simulink model "laba_2"  (R2020b)
settings: Solver=VariableStepAuto  StartTime=0.0  StopTime=15  RelTol=1e-3
settings Model: Creator=vak90  LastModifiedBy=Mi-Mi-Mishka
settings DebuggingCC: ArithmeticOperatorsInVariantConditions=warning
settings SFSimCC: CustomCodeUndefinedFunction=UseInterfaceOnly

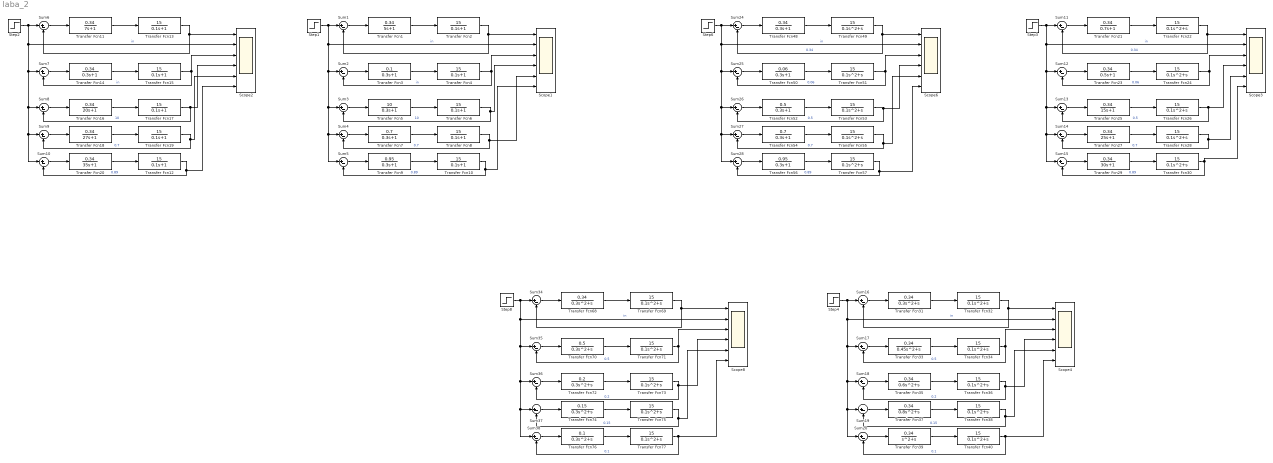
== system laba_2 ==
  Scope{1..4,6,8} (6 alike) : Scope  NumInputPorts=6
  Step{1..4,6,8} (6 alike) : Step  Time=0.1  SampleTime=0
  Sum{1..20,24..28,34..38} (30 alike) : Sum  Inputs=|+-
  Transfer Fcn1 : TransferFcn  Numerator=[0.34]  Denominator=[5 1]
  Transfer Fcn{2,4,6,8,10,12..13,15,17,19} (10 alike) : TransferFcn  Numerator=[15]  Denominator=[0.1 1 ]
  Transfer Fcn11 : TransferFcn  Numerator=[0.34]  Denominator=[7 1]
  Transfer Fcn14 : TransferFcn  Numerator=[0.34]  Denominator=[0.3 1]
  Transfer Fcn16 : TransferFcn  Numerator=[0.34]  Denominator=[20 1]
  Transfer Fcn18 : TransferFcn  Numerator=[0.34]  Denominator=[27 1]
  Transfer Fcn20 : TransferFcn  Numerator=[0.34]  Denominator=[35 1]
  Transfer Fcn21 : TransferFcn  Numerator=[0.34]  Denominator=[0.7 1]
  Transfer Fcn{22,24,26,28,30,32,34,36,38,40,49,51,53,55,57,69,71,73,75,77} (20 alike) : TransferFcn  Numerator=[15]  Denominator=[0.1 1 0]
  Transfer Fcn23 : TransferFcn  Numerator=[0.34]  Denominator=[0.5 1]
  Transfer Fcn25 : TransferFcn  Numerator=[0.34]  Denominator=[15 1]
  Transfer Fcn27 : TransferFcn  Numerator=[0.34]  Denominator=[25 1]
  Transfer Fcn29 : TransferFcn  Numerator=[0.34]  Denominator=[30 1]
  Transfer Fcn3 : TransferFcn  Numerator=[0.1]  Denominator=[0.3 1]
  Transfer Fcn31 : TransferFcn  Numerator=[0.34]  Denominator=[0.3 1 0]
  Transfer Fcn33 : TransferFcn  Numerator=[0.34]  Denominator=[0.45 1 0]
  Transfer Fcn35 : TransferFcn  Numerator=[0.34]  Denominator=[0.6 1 0]
  Transfer Fcn37 : TransferFcn  Numerator=[0.34]  Denominator=[0.8 1 0]
  Transfer Fcn39 : TransferFcn  Numerator=[0.34]  Denominator=[1 1 0]
  Transfer Fcn48 : TransferFcn  Numerator=[0.34]  Denominator=[0.3 1]
  Transfer Fcn5 : TransferFcn  Numerator=[10]  Denominator=[0.3 1]
  Transfer Fcn50 : TransferFcn  Numerator=[0.06]  Denominator=[0.3 1]
  Transfer Fcn52 : TransferFcn  Numerator=[0.5]  Denominator=[0.3 1]
  Transfer Fcn54 : TransferFcn  Numerator=[0.7]  Denominator=[0.3 1]
  Transfer Fcn56 : TransferFcn  Numerator=[0.95]  Denominator=[0.3 1]
  Transfer Fcn68 : TransferFcn  Numerator=[0.34]  Denominator=[0.3 1 0]
  Transfer Fcn7 : TransferFcn  Numerator=[0.7]  Denominator=[0.3 1]
  Transfer Fcn70 : TransferFcn  Numerator=[0.5]  Denominator=[0.3 1 0]
  Transfer Fcn72 : TransferFcn  Numerator=[0.2]  Denominator=[0.3 1 0]
  Transfer Fcn74 : TransferFcn  Numerator=[0.15]  Denominator=[0.3 1 0]
  Transfer Fcn76 : TransferFcn  Numerator=[0.1]  Denominator=[0.3 1 0]
  Transfer Fcn9 : TransferFcn  Numerator=[0.95]  Denominator=[0.3 1]
  wires:
  Step6/1 -> Sum28/1, Sum27/1, Sum26/1, Sum25/1, Scope6/2, Sum24/1  "in"
  Sum24/1 -> Transfer Fcn48/1
  Transfer Fcn48/1 -> Transfer Fcn49/1
  Transfer Fcn49/1 -> Sum24/2, Scope6/1  "0.34"
  Sum25/1 -> Transfer Fcn50/1
  Transfer Fcn50/1 -> Transfer Fcn51/1
  Sum26/1 -> Transfer Fcn52/1
  Transfer Fcn52/1 -> Transfer Fcn53/1
  Sum27/1 -> Transfer Fcn54/1
  Transfer Fcn54/1 -> Transfer Fcn55/1
  Sum28/1 -> Transfer Fcn56/1
  Transfer Fcn56/1 -> Transfer Fcn57/1
  Transfer Fcn51/1 -> Sum25/2, Scope6/3  "0.06"
  Transfer Fcn53/1 -> Scope6/4, Sum26/2  "0.5"
  Transfer Fcn55/1 -> Scope6/5, Sum27/2  "0.7"
  Transfer Fcn57/1 -> Scope6/6, Sum28/2  "0.89"
  Transfer Fcn68/1 -> Transfer Fcn69/1
  Transfer Fcn69/1 -> Sum34/2, Scope8/1
  Sum34/1 -> Transfer Fcn68/1
  Transfer Fcn73/1 -> Scope8/4, Sum36/2  "0.2"
  Step8/1 -> Sum38/1, Sum37/1, Sum36/1, Sum35/1, Scope8/2, Sum34/1  "in"
  Transfer Fcn71/1 -> Sum35/2, Scope8/3  "0.5"
  Transfer Fcn77/1 -> Scope8/6, Sum38/2  "0.1"
  Transfer Fcn75/1 -> Scope8/5, Sum37/2  "0.15"
  Sum35/1 -> Transfer Fcn70/1
  Transfer Fcn70/1 -> Transfer Fcn71/1
  Sum36/1 -> Transfer Fcn72/1
  Transfer Fcn72/1 -> Transfer Fcn73/1
  Sum37/1 -> Transfer Fcn74/1
  Transfer Fcn74/1 -> Transfer Fcn75/1
  Sum38/1 -> Transfer Fcn76/1
  Transfer Fcn76/1 -> Transfer Fcn77/1
  Sum4/1 -> Transfer Fcn7/1
  Transfer Fcn1/1 -> Transfer Fcn2/1
  Transfer Fcn3/1 -> Transfer Fcn4/1
  Transfer Fcn10/1 -> Scope1/6, Sum5/2  "0.89"
  Transfer Fcn2/1 -> Sum1/2, Scope1/1
  Transfer Fcn7/1 -> Transfer Fcn8/1
  Step1/1 -> Sum5/1, Sum4/1, Sum3/1, Sum2/1, Scope1/2, Sum1/1  "in"
  Transfer Fcn6/1 -> Scope1/4, Sum3/2  "10"
  Sum2/1 -> Transfer Fcn3/1
  Sum5/1 -> Transfer Fcn9/1
  Transfer Fcn8/1 -> Scope1/5, Sum4/2  "0.7"
  Sum3/1 -> Transfer Fcn5/1
  Sum1/1 -> Transfer Fcn1/1
  Transfer Fcn5/1 -> Transfer Fcn6/1
  Transfer Fcn9/1 -> Transfer Fcn10/1
  Transfer Fcn4/1 -> Sum2/2, Scope1/3  "in"
  Transfer Fcn20/1 -> Transfer Fcn12/1
  Transfer Fcn13/1 -> Sum6/2, Scope2/1
  Sum8/1 -> Transfer Fcn16/1
  Sum9/1 -> Transfer Fcn18/1
  Sum6/1 -> Transfer Fcn11/1
  Transfer Fcn16/1 -> Transfer Fcn17/1
  Sum7/1 -> Transfer Fcn14/1
  Transfer Fcn19/1 -> Scope2/5, Sum9/2  "0.7"
  Step2/1 -> Sum10/1, Sum9/1, Sum8/1, Sum7/1, Scope2/2, Sum6/1  "in"
  Sum10/1 -> Transfer Fcn20/1
  Transfer Fcn14/1 -> Transfer Fcn15/1
  Transfer Fcn12/1 -> Scope2/6, Sum10/2  "0.89"
  Transfer Fcn17/1 -> Scope2/4, Sum8/2  "10"
  Transfer Fcn18/1 -> Transfer Fcn19/1
  Transfer Fcn11/1 -> Transfer Fcn13/1
  Transfer Fcn15/1 -> Sum7/2, Scope2/3  "in"
  Sum15/1 -> Transfer Fcn29/1
  Transfer Fcn27/1 -> Transfer Fcn28/1
  Transfer Fcn29/1 -> Transfer Fcn30/1
  Transfer Fcn26/1 -> Sum13/2, Scope3/4  "0.5"
  Sum13/1 -> Transfer Fcn25/1
  Sum14/1 -> Transfer Fcn27/1
  Transfer Fcn23/1 -> Transfer Fcn24/1
  Transfer Fcn22/1 -> Sum11/2, Scope3/1  "0.34"
  Transfer Fcn30/1 -> Sum15/2, Scope3/6  "0.89"
  Transfer Fcn25/1 -> Transfer Fcn26/1
  Sum12/1 -> Transfer Fcn23/1
  Sum11/1 -> Transfer Fcn21/1
  Transfer Fcn28/1 -> Sum14/2, Scope3/5  "0.7"
  Transfer Fcn24/1 -> Sum12/2, Scope3/3  "0.06"
  Step3/1 -> Sum15/1, Sum14/1, Sum13/1, Sum12/1, Scope3/2, Sum11/1  "in"
  Transfer Fcn21/1 -> Transfer Fcn22/1
  Transfer Fcn36/1 -> Sum18/2, Scope4/4  "0.2"
  Sum16/1 -> Transfer Fcn31/1
  Sum19/1 -> Transfer Fcn37/1
  Sum18/1 -> Transfer Fcn35/1
  Transfer Fcn37/1 -> Transfer Fcn38/1
  Transfer Fcn32/1 -> Sum16/2, Scope4/1
  Sum20/1 -> Transfer Fcn39/1
  Transfer Fcn39/1 -> Transfer Fcn40/1
  Transfer Fcn34/1 -> Sum17/2, Scope4/3  "0.5"
  Transfer Fcn33/1 -> Transfer Fcn34/1
  Transfer Fcn40/1 -> Sum20/2, Scope4/6  "0.1"
  Transfer Fcn31/1 -> Transfer Fcn32/1
  Transfer Fcn35/1 -> Transfer Fcn36/1
  Transfer Fcn38/1 -> Scope4/5, Sum19/2  "0.15"
  Step4/1 -> Sum20/1, Sum19/1, Sum18/1, Sum17/1, Scope4/2, Sum16/1  "in"
  Sum17/1 -> Transfer Fcn33/1
